simulink model "ProblemNo_6"  (R2020b)
settings: Solver=VariableStepAuto  StartTime=0.0  StopTime=10.0  RelTol=1e-3
settings Model: Creator=Pavan  LastModifiedBy=Pavan

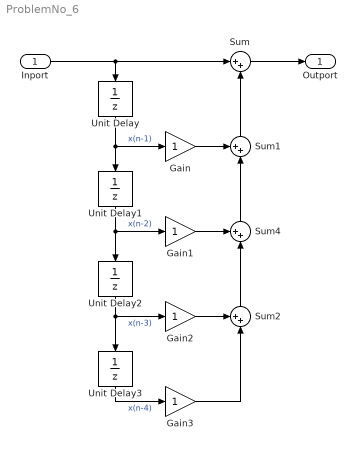
== system ProblemNo_6 ==
  Inport : Inport
  Gain{,1..3} (4 alike) : Gain
  Sum : Sum  Inputs=|++
  Sum1 : Sum  Inputs=++|
  Sum2 : Sum  Inputs=++|
  Sum4 : Sum  Inputs=++|
  Unit Delay{,1..3} (4 alike) : UnitDelay  SampleTime=-1  HasFrameUpgradeWarning=on
  Outport : Outport
  wires:
  Unit Delay/1 -> Unit Delay1/1, Gain/1  "x(n-1)"
  Inport/1 -> Sum/1, Unit Delay/1
  Unit Delay1/1 -> Unit Delay2/1, Gain1/1  "x(n-2)"
  Gain/1 -> Sum1/1
  Sum1/1 -> Sum/2
  Gain1/1 -> Sum4/1
  Sum4/1 -> Sum1/2
  Unit Delay2/1 -> Gain2/1, Unit Delay3/1  "x(n-3)"
  Gain2/1 -> Sum2/1
  Gain3/1 -> Sum2/2
  Unit Delay3/1 -> Gain3/1  "x(n-4)"
  Sum2/1 -> Sum4/2
  Sum/1 -> Outport/1
